simulink library "Environment_Lib"  (R2016b)
settings: Solver=ode45  StartTime=0.0  StopTime=10.0  RelTol=1e-3
values from neighbouring files (symbols this model uses):
  Env =     [UAV_modelconfig.mat]
undefined symbols (not defined in the file or in its folder): aeroassertmsg, F, Light, MIL
libraries: Environment_Lib x5, simulink x4, aerolibobsolete x2, aerolibconvert2 x2, aerolibwind2 x2, aerolibatmos2 x1, aerolibgravity2 x1, aerolibutil x1
settings Model: Creator=Paul Freeman  LastModifiedBy=UAVLAB
settings DataIOCC: LimitDataPoints=on  SaveFormat=Array  SignalLoggingSaveFormat=ModelDataLogs
settings OptimizationCC: BlockReduction=off  BooleanDataType=off  ExpressionDepthLimit=2147483647  LifeSpan=inf
settings DebuggingCC: SaveWithParameterizedLinksMsg=none  UnderspecifiedInitializationDetection=Classic  MergeDetectMultiDrivingBlocksExec=none  SignalResolutionControl=TryResolveAllWithWarning  FcnCallInpInsideContextMsg=warning  StateNameClashWarn=warning  StrictBusMsg=Warning  SFUnexpectedBacktrackingDiag=warning  SFNoUnconditionalDefaultTransitionDiag=warning  SFExecutionAtInitializationDiag=none
settings HardwareCC: ProdBitPerPointer=32  ProdBitPerSizeT=32  ProdBitPerPtrDiffT=32  ProdLargestAtomicFloat=None  ProdIntDivRoundTo=Undefined  ProdEndianess=Unspecified  ProdWordSize=32  ProdHWDeviceType=32-bit Generic  TargetUnknown=on
settings ModelReferenceCC: PropagateSignalLabelsOutOfModel=off
settings GRTTargetCC: TargetLangStandard=C89/C90 (ANSI)  GeneratePreprocessorConditionals=Disable all  CombineOutputUpdateFcns=off  GRTInterface=on
settings ConfigComp: CovMetricSettings=dw  CovHtmlReporting=on  CovSaveCumulativeToWorkspaceVar=on  CovSaveSingleToWorkspaceVar=on  CovExternalEMLEnable=off

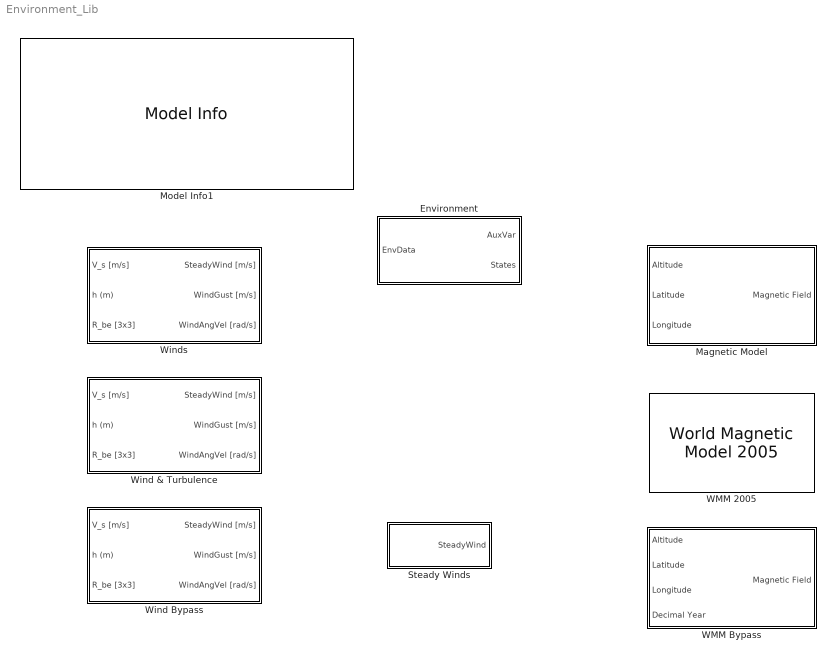
== system Environment_Lib ==
  Environment : Subsystem
  Magnetic Model : Subsystem  BlockChoice=WMM 2005
      settings: TemplateBlock=self  MemberBlocks=WMM 2005,WMM Bypass
  Model Info1 : simulink/Model-Wide Utilities/Model Info  BlockCM=None  Frame=on  DisplayStringWithTags=|  HorizontalTextAlignment=Left  LeftAlignmentValue=0.02  SourceBlockDiagram=Environment_Lib  TagMaxNumber=20
      | MODEL INFORMATION
      | Environment Library
      | 
      | University of Minnesota
      | Aerospace Engineering and Mechanics
      | Copyright 2011 Regents of the University of Minnesota. All rights reserved.
      | 
      | == SVN Info ==
      | Last modified by %<LastModifiedBy> on %<LastModificationDate>
  Steady Winds : Subsystem
  WMM 2005 : aerolibobsolete/World Magnetic Model 2005  units=Metric (MKS)  time_in=on  month=August  day=1  year=2009  action=None  h_out=off  dec_out=off  inc_out=off  ti_out=off
  WMM Bypass : Subsystem  AncestorBlock=aerolibgravity2/World Magnetic Model 2005  mask(World Magnetic Model 2005){units=Metric (MKS), time_in=on, month=August, day=1, year=2009, action=None, h_out=off, dec_out=off, inc_out=off, ti_out=off}
      mask prompts: time_in "Input decimal year"; action "Action for out of range input:"; h_out "Output horizontal intensity"; dec_out "Output declination"; inc_out "Output inclination"; ti_out "Output total intensity"
      mask help:
      | Calculate the Earth's magnetic field at a specific location and time using the World Magnetic Model (WMM). This model is valid for the year 2005 through the year 2010.
      |
      | The WMM-2005 can be found on the web at http://www.ngdc.noaa.gov/seg/WMM/DoDWMM.shtml and in "NOAA Technical Report: The US/UK World Magnetic Model for 2005-2010 ".
      |
      | Height is entered in length units of selected unit system. Latitude and longitude are entered in degrees.
      mask init:
      | [ports,dyear,maxdef,epoch,c,cd,fn,fm,snorm,k]=aeroicon('aeroblkwmm2005','icon');
      mask Help: eval('asbhelp');
      mask TypeOptions units: Metric (MKS) | English
      mask Callback time_in: aeroicon('aeroblkwmm');
      mask TypeOptions month: January | February | March | April | May | June | July | August | September | October | November | December
      mask Callback month: aeroicon('aeroblkwmm');
      mask TypeOptions day: 1 | 2 | 3 | 4 | 5 | 6 | 7 | 8 | 9 | 10 | 11 | 12 | 13 | 14 | 15 | 16 | 17 | 18 | 19 | 20 | 21 | 22 | 23 | 24 | 25 | 26 | 27 | 28 | 29 | 30 | 31
      mask Callback day: aeroicon('aeroblkwmm');
      mask TypeOptions year: 2005 | 2006 | 2007 | 2008 | 2009 | 2010
      mask Callback year: aeroicon('aeroblkwmm');
      mask TypeOptions action: None | Warning | Error
      mask Display:
      | port_label(ports(1).type,ports(1).port,ports(1).txt);
      | port_label(ports(2).type,ports(2).port,ports(2).txt,'texmode','on');
      | port_label(ports(3).type,ports(3).port,ports(3).txt,'texmode','on');
      | port_label(ports(4).type,ports(4).port,ports(4).txt);
      | port_label(ports(5).type,ports(5).port,ports(5).txt);
      | port_label(ports(6).type,ports(6).port,ports(6).txt);
      | port_label(ports(7).type,ports(7).port,ports(7).txt);
      | port_label(ports(8).type,ports(8).port,ports(8).txt);
      | port_label(ports(9).type,ports(9).port,ports(9).txt);
  Wind & Turbulence : Subsystem
  Wind Bypass : Subsystem
      settings: MinAlgLoopOccurrences=on
  Winds : Subsystem  BlockChoice=Wind & Turbulence
      settings: TemplateBlock=self  MemberBlocks=Wind & Turbulence,Wind Bypass

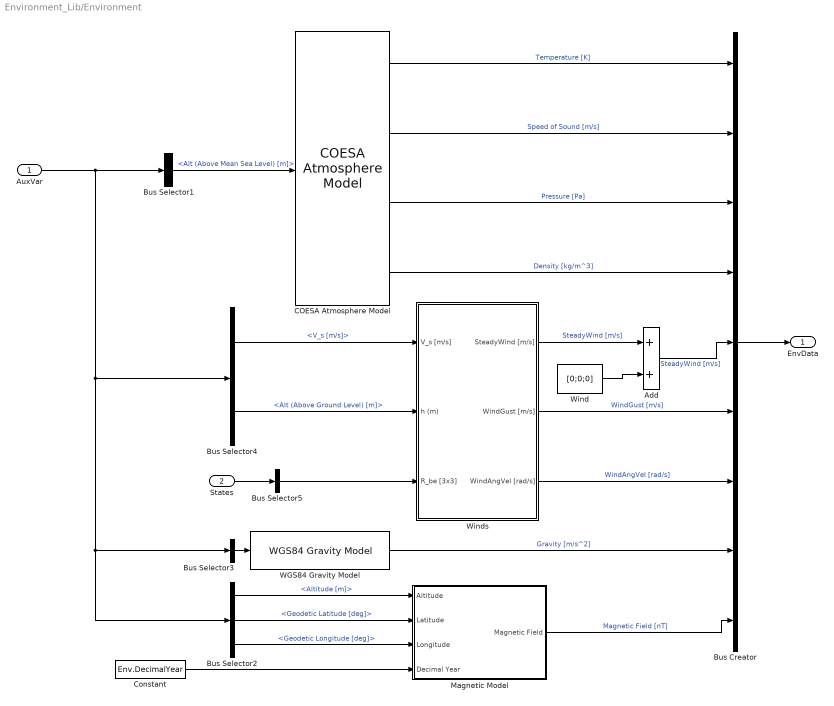
== system Environment_Lib/Environment ==
  AuxVar : Inport
  States : Inport  Port=2
  Add : Sum
  Bus Creator : BusCreator  Inputs=9
  Bus Selector1 : BusSelector  OutputSignals=Nav.Alt (Above Mean Sea Level) [m]
  Bus Selector2 : BusSelector  OutputSignals=Nav.Altitude [m],Nav.Geodetic Latitude [deg],Nav.Geodetic Longitude [deg]
  Bus Selector3 : BusSelector  OutputSignals=Nav.Geodetic Latitude [deg],Nav.Geodetic Longitude [deg],Nav.Altitude [m]  OutputAsBus=on
  Bus Selector4 : BusSelector  OutputSignals=WindAxesParam.V_s [m/s],Nav.Alt (Above Ground Level) [m]
  Bus Selector5 : BusSelector  OutputSignals=R_be [3x3]  OutputAsBus=on
  COESA Atmosphere Model : aerolibatmos2/COESA Atmosphere Model  units=Metric (MKS)  spec=1976 COESA-extended U.S. Standard Atmosphere  model=Profile  profile_var=High temperature  profile_percent=1%  profile_alt=5 km (16404 ft)  envelope_var=High temperature  envelope_percent=1%  action=Warning
  Constant : Constant  Value=Env.DecimalYear
  Magnetic Model : Subsystem  BlockChoice=WMM Bypass
      settings: AttributesFormatString=%<BlockChoice>  TemplateBlock=Environment_Lib/Magnetic Model  MemberBlocks=WMM 2005,WMM Bypass
  "WGS84 Gravity Model " : aerolibgravity2/WGS84 Gravity Model   model=WGS84 Taylor Series  units=Metric (MKS)  no_atmos=on  precessing=on  jd_loc=off  month=October  day=10  year=2004  no_centrifugal=on  action=Warning
  Wind : Constant  Value=[0;0;0]
  Winds : Subsystem  BlockChoice=Wind Bypass
      settings: AttributesFormatString=%<BlockChoice>  TemplateBlock=Environment_Lib/Winds  MemberBlocks=Wind & Turbulence,Wind Bypass
  EnvData : Outport
  wires:
  Bus Selector5/1 -> Winds/3(R_be [3x3])
  States/1 -> Bus Selector5/1
  AuxVar/1 -> Bus Selector1/1, Bus Selector4/1, Bus Selector3/1, Bus Selector2/1
  Wind/1 -> Add/2
  Add/1 -> Bus Creator/5  "SteadyWind [m/s]"
  Constant/1 -> Magnetic Model/4(Decimal Year)
  Bus Selector3/1 -> "WGS84 Gravity Model "/1
  Bus Selector2/3 -> Magnetic Model/3(Longitude)  "<Geodetic Longitude [deg]>"
  Bus Selector2/2 -> Magnetic Model/2(Latitude)  "<Geodetic Latitude [deg]>"
  Bus Selector2/1 -> Magnetic Model/1(Altitude)  "<Altitude [m]>"
  Magnetic Model/1(Magnetic Field) -> Bus Creator/9  "Magnetic Field [nT]"
  "WGS84 Gravity Model "/1 -> Bus Creator/8  "Gravity [m/s^2]"
  Winds/3(WindAngVel [rad/s]) -> Bus Creator/7  "WindAngVel [rad/s]"
  Winds/2(WindGust [m/s]) -> Bus Creator/6  "WindGust [m/s]"
  Winds/1(SteadyWind [m/s]) -> Add/1  "SteadyWind [m/s]"
  COESA Atmosphere Model/4 -> Bus Creator/4  "Density [kg/m^3]"
  COESA Atmosphere Model/1 -> Bus Creator/1  "Temperature [K]"
  COESA Atmosphere Model/2 -> Bus Creator/2  "Speed of Sound [m/s]"
  COESA Atmosphere Model/3 -> Bus Creator/3  "Pressure [Pa]"
  Bus Selector1/1 -> COESA Atmosphere Model/1  "<Alt (Above Mean Sea Level) [m]>"
  Bus Creator/1 -> EnvData/1
  Bus Selector4/1 -> Winds/1(V_s [m/s])  "<V_s [m/s]>"
  Bus Selector4/2 -> Winds/2(h (m))  "<Alt (Above Ground Level) [m]>"

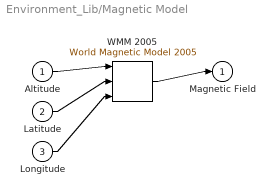
== system Environment_Lib/Magnetic Model ==
  Altitude : Inport
  Latitude : Inport  Port=2
  Longitude : Inport  Port=3
  WMM 2005 : aerolibobsolete/World Magnetic Model 2005  units=Metric (MKS)  time_in=off  month=August  day=1  year=2009  action=None  h_out=off  dec_out=off  inc_out=off  ti_out=off
  Magnetic Field : Outport
  wires:
  Altitude/1 -> WMM 2005/1
  Latitude/1 -> WMM 2005/2
  Longitude/1 -> WMM 2005/3
  WMM 2005/1 -> Magnetic Field/1

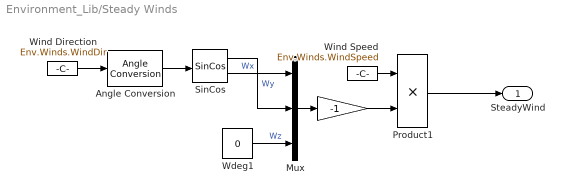
== system Environment_Lib/Steady Winds ==
  " " : Gain  Gain=-1  SaturateOnIntegerOverflow=on  OutDataTypeStr=Inherit: Same as input  ParamDataTypeStr=Inherit: Same as input
  Angle Conversion : aerolibconvert2/Angle Conversion  SystemSampleTime=-1  IU=deg  OU=rad
  Mux : Mux  Inputs=3
  Product1 : Product  SaturateOnIntegerOverflow=on  InputSameDT=on  OutDataTypeStr=Inherit: Same as first input
  SinCos : aerolibutil/SinCos  SystemSampleTime=-1
  Wdeg1 : Constant  Value=0  OutDataTypeStr=Inherit: Inherit via back propagation
  Wind Direction : Constant  Value=Env.Winds.WindDir  OutDataTypeStr=Inherit: Inherit via back propagation
  Wind Speed : Constant  Value=Env.Winds.WindSpeed  OutDataTypeStr=Inherit: Inherit via back propagation
  SteadyWind : Outport
  wires:
  " "/1 -> Product1/2
  Product1/1 -> SteadyWind/1
  Mux/1 -> " "/1
  Wdeg1/1 -> Mux/3  "Wz"
  Angle Conversion/1 -> SinCos/1
  SinCos/1 -> Mux/2  "Wy"
  SinCos/2 -> Mux/1  "Wx"
  Wind Speed/1 -> Product1/1
  Wind Direction/1 -> Angle Conversion/1

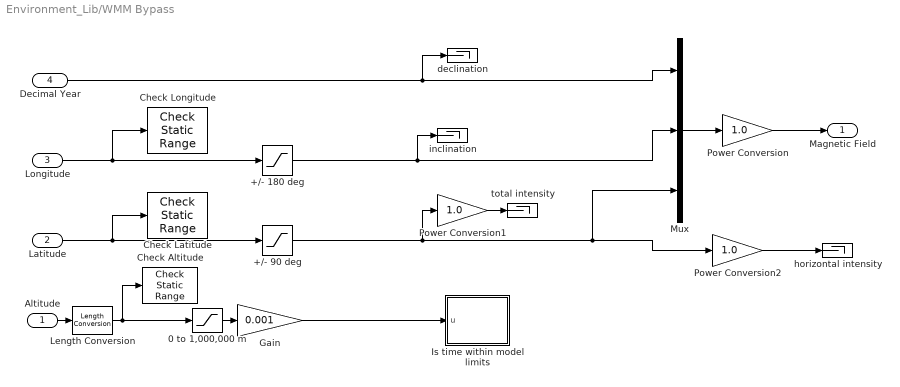
== system Environment_Lib/WMM Bypass ==
  Altitude : Inport
  Latitude : Inport  Port=2
  Longitude : Inport  Port=3
  Decimal Year : Inport  Port=4
  +/- 180 deg : Saturate  UpperLimit=180.0  LowerLimit=-180.0
  +/- 90 deg : Saturate  UpperLimit=90.0  LowerLimit=-90.0
  0 to 1,000,000 m : Saturate  UpperLimit=1000000.0  LowerLimit=0
  Check Altitude : simulink/Model Verification/Check  Static Range  Description=0 <= u <= 1000000  max=1000000  max_included=on  min=0  min_included=on  enabled=off  callback=aeroassertmsg('aeroblkwmm','alt','none')  stopWhenAssertionFail=off  export=off  icon=graphic
  Check Latitude : simulink/Model Verification/Check  Static Range  Description=-90 <= u <= 90  max=90  max_included=on  min=-90  min_included=on  enabled=off  callback=aeroassertmsg('aeroblkwmm','lat','none')  stopWhenAssertionFail=off  export=off  icon=graphic
  Check Longitude : simulink/Model Verification/Check  Static Range  Description=-180 <= u <= 180  max=180  max_included=on  min=-180  min_included=on  enabled=off  callback=aeroassertmsg('aeroblkwmm','lon','none')  stopWhenAssertionFail=off  export=off  icon=graphic
  Gain : Gain  Gain=0.001  SaturateOnIntegerOverflow=on  OutDataTypeStr=Inherit: Same as input  ParamDataTypeStr=Inherit: Same as input
  Is time within model limits : Subsystem  Description=0 <= u <= 5  mask(Checks_SRange){max=5, max_included=on, min=0, min_included=on, enabled=off, callback=aeroassertmsg('aeroblkwmm','time','none'), stopWhenAssertionFail=off, export=off, icon=graphic}
      mask prompts: max "Upper bound:"; max_included "Inclusive upper bound"; min "Lower bound:"; min_included "Inclusive lower bound"; enabled "Enable assertion"; callback "Simulation callback when assertion fails (optional):"; stopWhenAssertionFail "Stop simulation when assertion fails"; export "Output assertion signal"; icon "Select icon type:"
      mask help: Assert that the input signal lies between a static lower and upper bound or optionally equals either bound.
      mask init:
      | update_assert_sys(gcbh);
      mask TypeOptions icon: graphic | text
      mask Display:
      | image(imread('Checks_SRange.bmp','bmp'),'center')
      | plot([0 1], [0 1]);
      | plot([0 1],[1 0]);
  Length Conversion : aerolibconvert2/Length Conversion  IU=m  OU=m
  Mux : Mux  Inputs=3
  Power Conversion : Gain  Gain=1.0  SaturateOnIntegerOverflow=on  OutDataTypeStr=Inherit: Same as input  ParamDataTypeStr=Inherit: Same as input
  Power Conversion1 : Gain  Gain=1.0  SaturateOnIntegerOverflow=on  OutDataTypeStr=Inherit: Same as input  ParamDataTypeStr=Inherit: Same as input
  Power Conversion2 : Gain  Gain=1.0  SaturateOnIntegerOverflow=on  OutDataTypeStr=Inherit: Same as input  ParamDataTypeStr=Inherit: Same as input
  declination : Terminator
  horizontal intensity : Terminator
  inclination : Terminator
  total intensity : Terminator
  Magnetic Field : Outport
  wires:
  Altitude/1 -> Length Conversion/1
  Length Conversion/1 -> 0 to 1,000,000 m/1, Check Altitude/1
  Decimal Year/1 -> declination/1, Mux/1
  Latitude/1 -> +/- 90 deg/1, Check Latitude/1
  Longitude/1 -> +/- 180 deg/1, Check Longitude/1
  Gain/1 -> Is time within model limits/1(u)
  Mux/1 -> Power Conversion/1
  Power Conversion/1 -> Magnetic Field/1
  Power Conversion1/1 -> total intensity/1
  Power Conversion2/1 -> horizontal intensity/1
  +/- 90 deg/1 -> Power Conversion1/1, Power Conversion2/1, Mux/3
  +/- 180 deg/1 -> inclination/1, Mux/2
  0 to 1,000,000 m/1 -> Gain/1

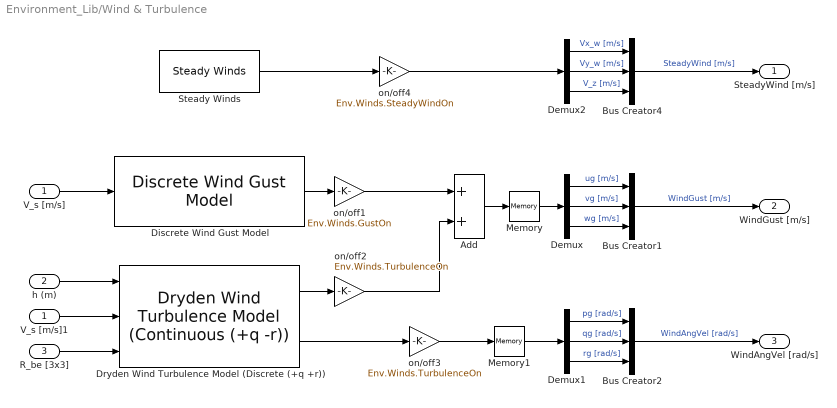
== system Environment_Lib/Wind & Turbulence ==
  V_s [m/s] : Inport
  h (m) : Inport  Port=2
  R_be [3x3] : Inport  Port=3
  Add : Sum
  Bus Creator1 : BusCreator  Inputs=3
  Bus Creator2 : BusCreator  Inputs=3
  Bus Creator4 : BusCreator  Inputs=3
  Demux : Demux  Outputs=3
  Demux1 : Demux  Outputs=3
  Demux2 : Demux  Outputs=3
  Discrete Wind Gust Model : aerolibwind2/Discrete Wind Gust Model  units=Metric (MKS)  Gx=on  Gy=on  Gz=on  t_0=Env.Winds.GustStartTime  d_m=Env.Winds.GustLength  v_m=Env.Winds.GustAmplitude
  Dryden Wind Turbulence Model (Discrete (+q +r)) : aerolibwind2/Dryden Wind Turbulence Model  (Continuous (+q -r))  units=Metric (MKS)  spec=MIL-F-8785C  model=Discrete Dryden (+q +r)  W20=Env.Winds.TurbWindSpeed  Wdeg=Env.Winds.TurbWindDir  TurbProb=10^-2 - Light  L_high=762  Wingspan=AC.Geometry.b  ts=SampleTime  Seed=[23341 23342 23343 23344]  T_on=on
  Memory : Memory
  Memory1 : Memory
  Steady Winds : Environment_Lib/Steady Winds
  V_s [m/s]1 : InportShadow
  on/off1 : Gain  Gain=Env.Winds.GustOn
  on/off2 : Gain  Gain=Env.Winds.TurbulenceOn
  on/off3 : Gain  Gain=Env.Winds.TurbulenceOn
  on/off4 : Gain  Gain=Env.Winds.SteadyWindOn
  SteadyWind [m/s] : Outport
  WindGust [m/s] : Outport  Port=2
  WindAngVel [rad/s] : Outport  Port=3
  wires:
  Demux/1 -> Bus Creator1/1  "ug [m/s]"
  Demux1/3 -> Bus Creator2/3  "rg [rad/s]"
  Demux1/2 -> Bus Creator2/2  "qg [rad/s]"
  Demux1/1 -> Bus Creator2/1  "pg [rad/s]"
  Demux/3 -> Bus Creator1/3  "wg [m/s]"
  Demux/2 -> Bus Creator1/2  "vg [m/s]"
  V_s [m/s]/1 -> Discrete Wind Gust Model/1
  Demux2/1 -> Bus Creator4/1  "Vx_w [m/s]"
  Demux2/3 -> Bus Creator4/3  "V_z [m/s]"
  Demux2/2 -> Bus Creator4/2  "Vy_w [m/s]"
  Steady Winds/1 -> on/off4/1
  Add/1 -> Memory/1
  Discrete Wind Gust Model/1 -> on/off1/1
  Dryden Wind Turbulence Model (Discrete (+q +r))/1 -> on/off2/1
  on/off3/1 -> Memory1/1
  on/off4/1 -> Demux2/1
  on/off1/1 -> Add/1
  on/off2/1 -> Add/2
  Memory/1 -> Demux/1
  Memory1/1 -> Demux1/1
  Bus Creator4/1 -> SteadyWind [m/s]/1  "SteadyWind [m/s]"
  Bus Creator1/1 -> WindGust [m/s]/1  "WindGust [m/s]"
  Bus Creator2/1 -> WindAngVel [rad/s]/1  "WindAngVel [rad/s]"
  Dryden Wind Turbulence Model (Discrete (+q +r))/2 -> on/off3/1
  R_be [3x3]/1 -> Dryden Wind Turbulence Model (Discrete (+q +r))/3
  h (m)/1 -> Dryden Wind Turbulence Model (Discrete (+q +r))/1
  V_s [m/s]1/1 -> Dryden Wind Turbulence Model (Discrete (+q +r))/2

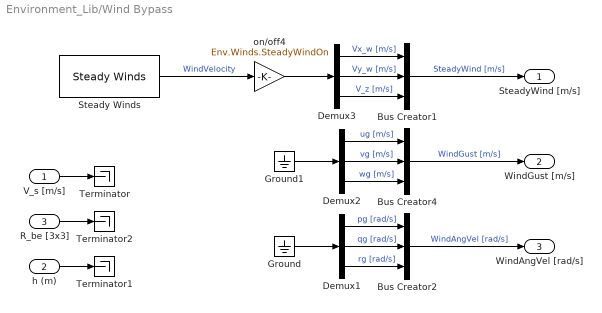
== system Environment_Lib/Wind Bypass ==
  V_s [m/s] : Inport
  h (m) : Inport  Port=2
  R_be [3x3] : Inport  Port=3
  Bus Creator1 : BusCreator  Inputs=3
  Bus Creator2 : BusCreator  Inputs=3
  Bus Creator4 : BusCreator  Inputs=3
  Demux1 : Demux  Outputs=3
  Demux2 : Demux  Outputs=3
  Demux3 : Demux  Outputs=3
  Ground : Ground
  Ground1 : Ground
  Steady Winds : Environment_Lib/Steady Winds
  Terminator : Terminator
  Terminator1 : Terminator
  Terminator2 : Terminator
  on/off4 : Gain  Gain=Env.Winds.SteadyWindOn
  SteadyWind [m/s] : Outport
  WindGust [m/s] : Outport  Port=2
  WindAngVel [rad/s] : Outport  Port=3
  wires:
  Demux1/3 -> Bus Creator2/3  "rg [rad/s]"
  Demux1/2 -> Bus Creator2/2  "qg [rad/s]"
  Demux1/1 -> Bus Creator2/1  "pg [rad/s]"
  Steady Winds/1 -> on/off4/1  "WindVelocity"
  V_s [m/s]/1 -> Terminator/1
  Ground/1 -> Demux1/1
  Demux2/1 -> Bus Creator4/1  "ug [m/s]"
  Demux2/3 -> Bus Creator4/3  "wg [m/s]"
  Demux2/2 -> Bus Creator4/2  "vg [m/s]"
  Ground1/1 -> Demux2/1
  Demux3/1 -> Bus Creator1/1  "Vx_w [m/s]"
  Demux3/3 -> Bus Creator1/3  "V_z [m/s]"
  Demux3/2 -> Bus Creator1/2  "Vy_w [m/s]"
  on/off4/1 -> Demux3/1
  Bus Creator1/1 -> SteadyWind [m/s]/1  "SteadyWind [m/s]"
  Bus Creator4/1 -> WindGust [m/s]/1  "WindGust [m/s]"
  Bus Creator2/1 -> WindAngVel [rad/s]/1  "WindAngVel [rad/s]"
  R_be [3x3]/1 -> Terminator2/1
  h (m)/1 -> Terminator1/1

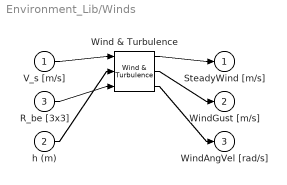
== system Environment_Lib/Winds ==
  V_s [m/s] : Inport
  h (m) : Inport  Port=2
  R_be [3x3] : Inport  Port=3
  Wind & Turbulence : Environment_Lib/Wind & Turbulence
  SteadyWind [m/s] : Outport
  WindGust [m/s] : Outport  Port=2
  WindAngVel [rad/s] : Outport  Port=3
  wires:
  V_s [m/s]/1 -> Wind & Turbulence/1
  h (m)/1 -> Wind & Turbulence/2
  R_be [3x3]/1 -> Wind & Turbulence/3
  Wind & Turbulence/1 -> SteadyWind [m/s]/1
  Wind & Turbulence/2 -> WindGust [m/s]/1
  Wind & Turbulence/3 -> WindAngVel [rad/s]/1

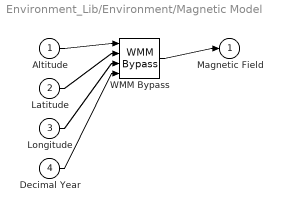
== system Environment_Lib/Environment/Magnetic Model ==
  Altitude : Inport
  Latitude : Inport  Port=2
  Longitude : Inport  Port=3
  Decimal Year : Inport  Port=4
  WMM Bypass : Environment_Lib/WMM Bypass  units=Metric (MKS)  time_in=on  month=August  day=1  year=2009  action=None  h_out=off  dec_out=off  inc_out=off  ti_out=off
  Magnetic Field : Outport
  wires:
  WMM Bypass/1 -> Magnetic Field/1
  Decimal Year/1 -> WMM Bypass/4
  Longitude/1 -> WMM Bypass/3
  Latitude/1 -> WMM Bypass/2
  Altitude/1 -> WMM Bypass/1

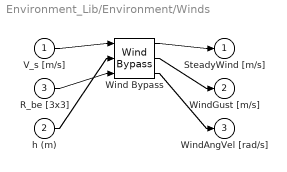
== system Environment_Lib/Environment/Winds ==
  V_s [m/s] : Inport
  h (m) : Inport  Port=2
  R_be [3x3] : Inport  Port=3
  Wind Bypass : Environment_Lib/Wind Bypass
  SteadyWind [m/s] : Outport
  WindGust [m/s] : Outport  Port=2
  WindAngVel [rad/s] : Outport  Port=3
  wires:
  Wind Bypass/3 -> WindAngVel [rad/s]/1
  Wind Bypass/2 -> WindGust [m/s]/1
  Wind Bypass/1 -> SteadyWind [m/s]/1
  R_be [3x3]/1 -> Wind Bypass/3
  h (m)/1 -> Wind Bypass/2
  V_s [m/s]/1 -> Wind Bypass/1

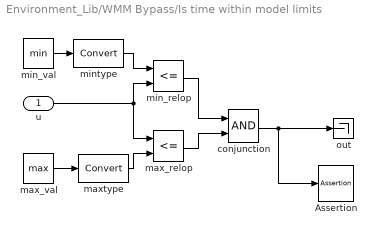
== system Environment_Lib/WMM Bypass/Is time within model limits ==
  u : Inport
  Assertion : Assertion  Enabled=off  AssertionFailFcn=evalin('base',callback)  StopWhenAssertionFail=off
  conjunction : Logic
  max_relop : RelationalOperator  Operator=<=  RndMeth=Nearest  InputSameDT=on
  max_val : Constant  Value=max
  maxtype : DataTypeConversion  SaturateOnIntegerOverflow=on  RndMeth=Zero
  min_relop : RelationalOperator  Operator=<=  RndMeth=Nearest  InputSameDT=on
  min_val : Constant  Value=min
  mintype : DataTypeConversion  SaturateOnIntegerOverflow=on  RndMeth=Zero
  out : Terminator
  wires:
  maxtype/1 -> max_relop/2
  mintype/1 -> min_relop/1
  conjunction/1 -> Assertion/1, out/1
  max_relop/1 -> conjunction/2
  min_relop/1 -> conjunction/1
  max_val/1 -> maxtype/1
  min_val/1 -> mintype/1
  u/1 -> max_relop/1, min_relop/2
